simulink model "task4"  (R2016b)
settings: Solver=VariableStepAuto  StartTime=0.0  StopTime=10.0  RelTol=1e-3
values from neighbouring files (symbols this model uses):
  eta_0 = [1.95 0.05 0]'    [task4_init.m]
  eta_d_0 = [2 0 0]'    [task4_init.m]
  eta_d_1 = [10 4 0]'    [task4_init.m]
  s_0 = 0    [task4_init.m]
  U_ref = 0.5    [task4_init.m]
settings Model: Creator=Ørjan  LastModifiedBy=Ørjan

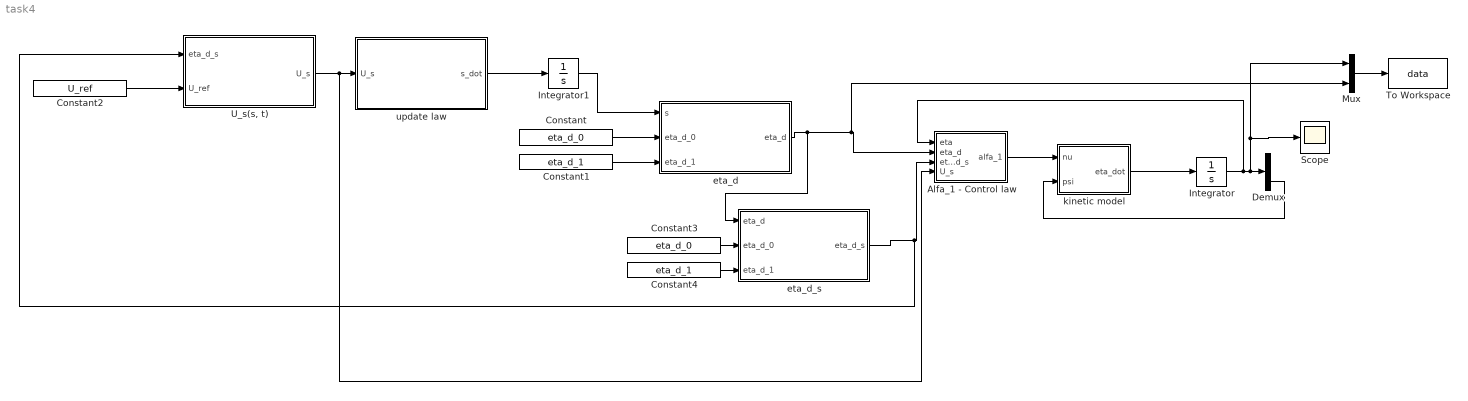
== system task4 ==
  Alfa_1 - Control law : MATLAB Function  TreatAsAtomicUnit=on
  Constant : Constant  Value=eta_d_0
  Constant1 : Constant  Value=eta_d_1
  Constant2 : Constant  Value=U_ref
  Constant3 : Constant  Value=eta_d_0
  Constant4 : Constant  Value=eta_d_1
  Demux : Demux  Outputs=3
  Integrator : Integrator  InitialCondition=eta_0
  Integrator1 : Integrator  InitialCondition=s_0
  Mux : Mux  Inputs=2
  Scope : Scope
  To Workspace : ToWorkspace  VariableName=data  SampleTime=-1
  "U_s(s, t)" : MATLAB Function  TreatAsAtomicUnit=on
  eta_d : MATLAB Function  TreatAsAtomicUnit=on
  eta_d_s : MATLAB Function  TreatAsAtomicUnit=on
  kinetic model : MATLAB Function  TreatAsAtomicUnit=on
  update law : MATLAB Function  TreatAsAtomicUnit=on
  wires:
  kinetic model/1(eta_dot) -> Integrator/1
  Integrator/1 -> Alfa_1 - Control law/1(eta), Scope/1, Mux/1, Demux/1
  Demux/3 -> kinetic model/2(psi)
  Alfa_1 - Control law/1(alfa_1) -> kinetic model/1(nu)
  update law/1(s_dot) -> Integrator1/1
  Integrator1/1 -> eta_d/1(s)
  eta_d/1(eta_d) -> eta_d_s/1(eta_d), Mux/2, Alfa_1 - Control law/2(eta_d)
  eta_d_s/1(eta_d_s) -> "U_s(s, t)"/1(eta_d_s), Alfa_1 - Control law/3(eta_d_s)
  Mux/1 -> To Workspace/1
  Constant2/1 -> "U_s(s, t)"/2(U_ref)
  Constant/1 -> eta_d/2(eta_d_0)
  Constant1/1 -> eta_d/3(eta_d_1)
  Constant3/1 -> eta_d_s/2(eta_d_0)
  Constant4/1 -> eta_d_s/3(eta_d_1)
  "U_s(s, t)"/1(U_s) -> Alfa_1 - Control law/4(U_s), update law/1(U_s)

== matlab function task4/Alfa_1 - Control law ==
  data: eta input; alfa_1 output; eta_d input; eta_d_s input; U_s input
function alfa_1 = fcn(eta, eta_d, eta_d_s, U_s)
K_p = diag([0.2 0.2 0.1]);

psi = eta(3);
z_1 = [cos(psi) -sin(psi) 0; sin(psi) cos(psi) 0; 0 0 1]'*(eta-eta_d);
alfa_1 = -K_p*z_1 + eta_d_s*U_s;
end

== matlab function task4/kinetic model ==
  data: nu input; eta_dot output; psi input
function eta_dot  = R_psi(nu, psi)
eta_dot = [cos(psi) -sin(psi) 0; sin(psi) cos(psi) 0; 0 0 1]*nu;
end

== matlab function task4/U_s(s, t) ==
  data: U_s output; eta_d_s input; U_ref input
function U_s = U_s(eta_d_s, U_ref)
U_s = abs(U_ref)/sqrt(eta_d_s(1)^2+eta_d_s(2)^2);
end

== matlab function task4/eta_d_s ==
  data: eta_d_s output; eta_d input; eta_d_0 input; eta_d_1 input
function eta_d_s = eta_d_s(eta_d, eta_d_0, eta_d_1)
x_d_s = eta_d_1(1) - eta_d_0(1);
y_d_s = eta_d_1(2) - eta_d_0(2);
psi_d_s = (y_d_s*eta_d(1) - eta_d(2)*x_d_s)/(eta_d(1)^2 + eta_d(2)^2);
eta_d_s = [x_d_s;y_d_s; psi_d_s];
end

== matlab function task4/eta_d ==
  data: eta_d output; s input; eta_d_0 input; eta_d_1 input
function eta_d = eta_d(s, eta_d_0, eta_d_1)
eta_d = [0 0 0]';
x_d = (eta_d_1(1) - eta_d_0(1))*s + eta_d_0(1);
y_d = (eta_d_1(2) - eta_d_0(2))*s + eta_d_0(2);
psi_d = atan(y_d/x_d);
eta_d = [x_d; y_d; psi_d];
end

== matlab function task4/update law ==
  data: s_dot output; U_s input
function s_dot = s_dot(U_s)
s_dot = U_s;
end
